simulink model "SWC_IOEXP_type"  (R2021b)
settings: Solver=FixedStepDiscrete  StartTime=0.0  StopTime=10.0  RelTol=1e-3
settings Model: DataDictionary=APPTypes.sldd  Creator=FVT23010  LastModifiedBy=FVT23010
settings DataIOCC: SaveFormat=StructureWithTime
settings OptimizationCC: DefaultParameterBehavior=Inlined  EnhancedBackFolding=on  PassReuseOutputArgsAs=Individual arguments  ZeroExternalMemoryAtStartup=off  ZeroInternalMemoryAtStartup=off  OptimizeBlockOrder=speed  DifferentSizesBufferReuse=on  OptimizationCustomize=off  EfficientTunableParamExpr=on
settings DebuggingCC: ParameterTunabilityLossMsg=error
settings SFSimCC: MATLABDynamicMemAlloc=off
settings RTWCC: Description=AUTOSAR  SystemTargetFile=autosar.tlc  GenCodeOnly=on  TemplateMakefile=ert_default_tmf
settings CodeAppCC: ForceParamTrailComments=on  IgnoreCustomStorageClasses=off  OperatorAnnotations=on  SimulinkDataObjDesc=on  SFDataObjDesc=on  InsertBlockDesc=on
settings STFCustomTargetCC: TargetLangStandard=C99 (ISO)  MultiwordLength=256  ParMdlRefBuildCompliant=on  CompOptLevelCompliant=on  IncludeMdlTerminateFcn=off  CombineOutputUpdateFcns=on  SuppressErrorStatus=on  ERTCustomFileBanners=on  SupportNonFinite=off  SupportComplex=off  SupportContinuousTime=off  SupportNonInlinedSFcns=off  RemoveResetFunc=on  MATLABClassNameForMDSCustomization=Simulink.SoftwareTarget.ERTCustomization  AutosarCompliant=on  GRTInterface=off  UseToolchainInfoCompliant=on  LookupTableObjectStructAxisOrder=2,1,3,4,...  LUTObjectStructOrderEvenSpacing=Size,Table,Breakpoints  SystemTargetFile=autosar.tlc
settings ERTTargetCC: TargetLangStandard=C99 (ISO)  ConcurrentExecutionCompliant=off  IncludeMdlTerminateFcn=off  SuppressErrorStatus=on  SupportNonFinite=off  SupportComplex=off  ModelStepFunctionPrototypeControlCompliant=off  CPPClassGenCompliant=off  AutosarCompliant=on  LookupTableObjectStructAxisOrder=2,1,3,4,...  LUTObjectStructOrderEvenSpacing=Size,Table,Breakpoints  InlinedParameterPlacement=NonHierarchical  ERTCustomFileTemplate=example_file_process.tlc

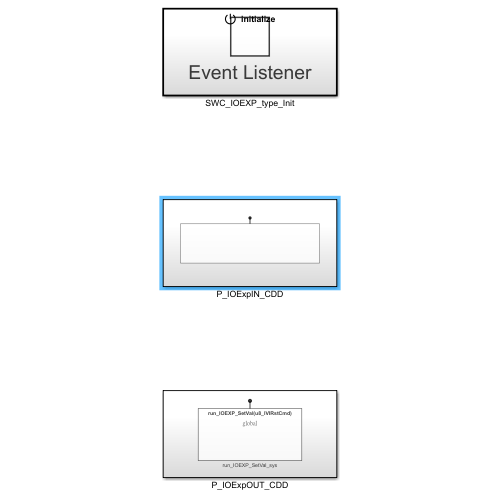
[thumbnail: Simulink's stored preview of the top-level diagram]
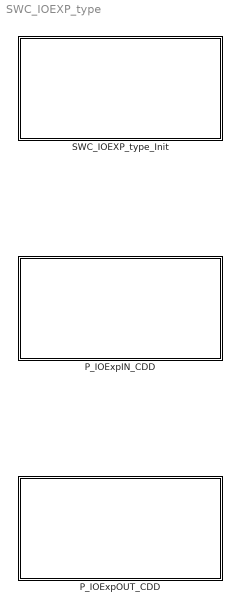
== system SWC_IOEXP_type ==
  P_IOExpIN_CDD : Subsystem
  P_IOExpOUT_CDD : Subsystem
  SWC_IOEXP_type_Init : Subsystem

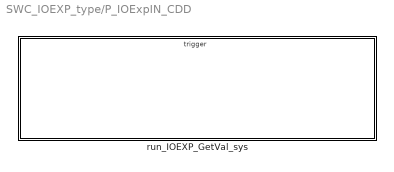
== system SWC_IOEXP_type/P_IOExpIN_CDD ==
  run_IOEXP_GetVal_sys : Subsystem

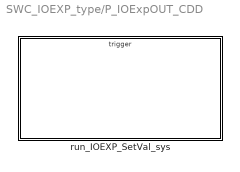
== system SWC_IOEXP_type/P_IOExpOUT_CDD ==
  run_IOEXP_SetVal_sys : Subsystem

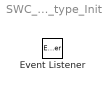
== system SWC_IOEXP_type/SWC_IOEXP_type_Init ==
  Event Listener : EventListener  EventName=reset

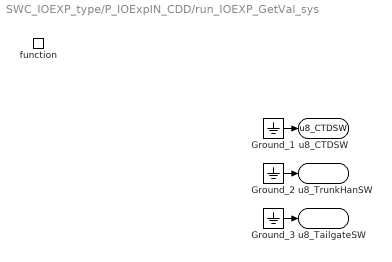
== system SWC_IOEXP_type/P_IOExpIN_CDD/run_IOEXP_GetVal_sys ==
  function : TriggerPort  TriggerType=function-call  IsSimulinkFunction=on  FunctionName=run_IOEXP_GetVal  VariantControl=(inherit)
  Ground_1 : Ground
  Ground_2 : Ground
  Ground_3 : Ground
  u8_CTDSW : ArgOut  OutDataTypeStr=uint8  ArgumentName=u8_CTDSW
  u8_TrunkHanSW : ArgOut  Port=2  OutDataTypeStr=uint8  ArgumentName=u8_TrunkHanSW
  u8_TailgateSW : ArgOut  Port=3  OutDataTypeStr=uint8  ArgumentName=u8_TailgateSW
  wires:
  Ground_1/1 -> u8_CTDSW/1
  Ground_2/1 -> u8_TrunkHanSW/1
  Ground_3/1 -> u8_TailgateSW/1

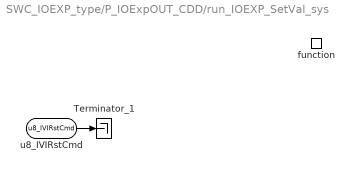
== system SWC_IOEXP_type/P_IOExpOUT_CDD/run_IOEXP_SetVal_sys ==
  function : TriggerPort  TriggerType=function-call  IsSimulinkFunction=on  FunctionName=run_IOEXP_SetVal  VariantControl=(inherit)
  Terminator_1 : Terminator
  u8_IVIRstCmd : ArgIn  OutDataTypeStr=uint8  ArgumentName=u8_IVIRstCmd
  wires:
  u8_IVIRstCmd/1 -> Terminator_1/1
